simulink model "RobotBody"  (R2024b)
settings: Solver=VariableStepAuto  StartTime=0.0  StopTime=5  RelTol=1e-3
values from neighbouring files (symbols this model uses):
  N = 20    [Init.m]
  s = U_weight*eye(InputNum)    [Init.m]
undefined symbols (not defined in the file or in its folder): DiscIntNeverNeededParam, X, Y, Z
libraries: sm_lib x306, nesl_utility x75, slpidlib x6, SignalEditorBlockLib x1
(part 1 of 7)
settings Model: Creator=Rengar  LastModifiedBy=ASUS
settings RTWCC: GPUComputeCapability=3.5

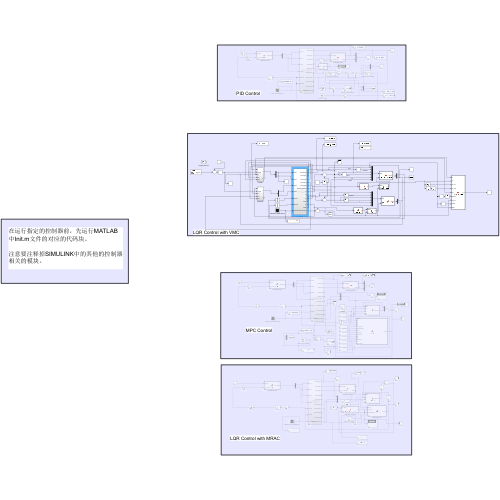
[thumbnail: Simulink's stored preview of the top-level diagram]
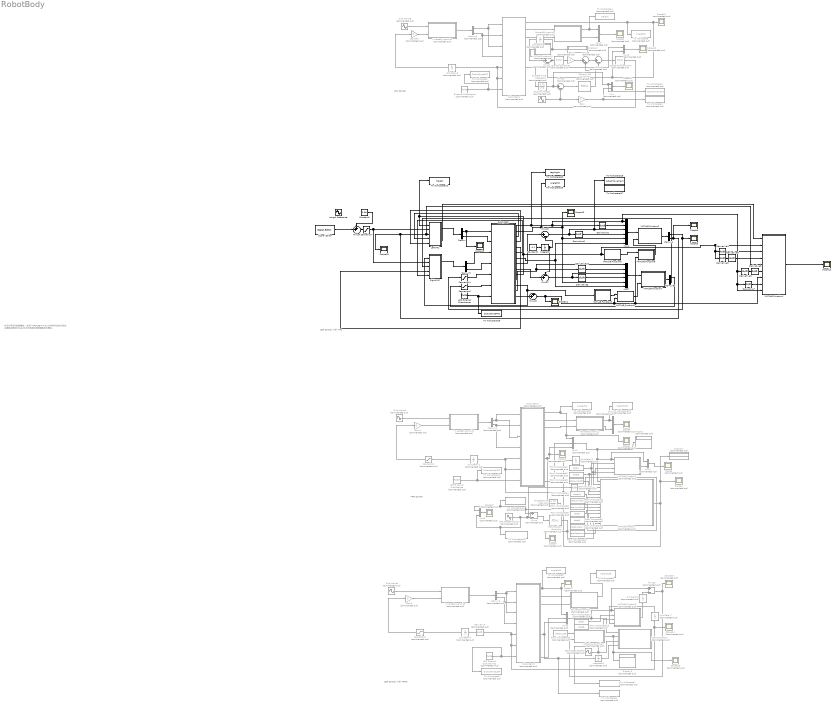
== system RobotBody ==
  note: 在运行指定的控制器前，先运行MATLAB中Init.m文件的对应的代码块。
      |
      | 注意要注释掉SIMULINK中的其他的控制器相关的模块。
  note: PID Control
  note: LQR Control with VMC
  note: MPC Control
  note: LQR Control with MRAC
  Adaptive controller1 : MATLAB Function  Commented=on  TreatAsAtomicUnit=on  SystemSampleTime=0.001
  Angle PID Controller : slpidlib/PID Controller  Commented=on  Controller=PID  Form=Parallel  TimeDomain=Continuous-time  UseExternalTs=off  SampleTime=-1  IntegratorMethod=Forward Euler  FilterMethod=Forward Euler  ControllerParametersSource=internal  P=1000  I=0  UseKiTs=off  D=500  UseExternalDerivativeSource=off  N=100  UseFilter=on  TunerSelectOption=Transfer Function Based (PID Tuner App)  InitialConditionSource=internal  InitialConditionForIntegrator=0  InitialConditionForFilter=0  DifferentiatorICPrevScaledInput=0  ExternalReset=none  TrackingMode=off  Kt=1  LimitOutput=off  SatLimitsSource=internal  UpperSaturationLimit=inf  LowerSaturationLimit=-inf  LinearizeAsGain=on  AntiWindupMode=none  Kb=1  LimitIntegrator=off  UpperIntegratorSaturationLimit=inf  LowerIntegratorSaturationLimit=-inf  POutMin=[]  POutMax=[]  IOutMin=[]  IOutMax=[]  DOutMin=[]  DOutMax=[]  NOutMin=[]  NOutMax=[]  SumOutMin=[]  SumOutMax=[]  SaturationOutMin=[]  SaturationOutMax=[]  PParamMin=[]  PParamMax=[]  IParamMin=[]  IParamMax=[]  DParamMin=[]  DParamMax=[]  NParamMin=[]  NParamMax=[]  KbParamMin=[]  KbParamMax=[]  KtParamMin=[]  KtParamMax=[]  KbOutMin=[]  KbOutMax=[]  KtOutMin=[]  KtOutMax=[]  IntegratorOutMin=[]  IntegratorOutMax=[]  FilterOutMin=[]  FilterOutMax=[]  SumI1OutMin=[]  SumI1OutMax=[]  SumI2OutMin=[]  SumI2OutMax=[]  SumI3OutMin=[]  SumI3OutMax=[]  SumI4OutMin=[]  SumI4OutMax=[]  SumDOutMin=[]  SumDOutMax=[]  DifferentiatorOutMin=[]  DifferentiatorOutMax=[]  FilterDiffOutCoefMin=[]  FilterDiffOutCoefMax=[]  ReciprocalOutMin=[]  ReciprocalOutMax=[]  SumDenOutMin=[]  SumDenOutMax=[]  SumNumOutMin=[]  SumNumOutMax=[]  DivideOutMin=[]  DivideOutMax=[]  UdiffTsProdOutMin=[]  UdiffTsProdOutMax=[]  NTsProdOutMin=[]  NTsProdOutMax=[]  UintegralTsProdOutMin=[]  UintegralTsProdOutMax=[]  UngainTsProdOutMin=[]  UngainTsProdOutMax=[]  ClampingZeroOutDataTypeStr=Inherit: Inherit via back propagation  ClampingZeroOutMin=[]  ClampingZeroOutMax=[]  FilterDenConstantOutDataTypeStr=Inherit: Inherit via back propagation  FilterDenConstantOutMin=[]  FilterDenConstantOutMax=[]  PCopyOutDataTypeStr=Inherit: Inherit via back propagation  PCopyOutMin=[]  PCopyOutMax=[]  NCopyOutDataTypeStr=Inherit: Inherit via back propagation  NCopyOutMin=[]  NCopyOutMax=[]  IntegratorContinuousStateAttributes=''  IntegratorStateMustResolveToSignalObject=off  IntegratorRTWStateStorageClass=Auto  FilterContinuousStateAttributes=''  FilterStateMustResolveToSignalObject=off  FilterRTWStateStorageClass=Auto  ParallelPVariant=InternalParameters  IdealPVariant=Disabled  IVariant=InternalParameters  DVariant=InternalParameters  IntegratorVariant=Continuous  SatVariant=Disabled  AWVariant=Passthrough  PCopyVariant=Disabled  TRVariant=Disabled  FdbkBlocksVariant=Forward  IdealPFdbkVariant=Disabled  SatFdbkVariant=Disabled  DerivativeFilterVariant=ContFilter  NVariant=InternalParameters  NCopyVariant=Disabled  FilterICVariant=InternalICsFilter  IntegratorICVariant=InternalICs  ExternalResetVariant=Disabled  TRSumVariant=Passthrough  SumFdbkVariant=Disabled  SumVariant=Sum_PID  TsampFilterVariant=InternalTs  TsampNgainVariant=Passthrough  TsampIntegralVariant=Disabled_SignalSpec  ExternalSaturationOutDataTypeStr=Inherit: Same as second input  DerivativeSourceVariant=ErrorSignal  PreIntVariant=InternalPreInt
  Constant1 : Constant  Value=0.06
  Constant2 : Constant  Value=-1.1
  Demux{,4..6} (4 alike) : Demux  Outputs=2
  Demux1 : Demux  Commented=on  Outputs=2
  Demux2 : Demux  Commented=on  Outputs=2
  Demux3 : Demux  Commented=on  Outputs=2
  Derivative : Derivative  Commented=on
  Derivative{1..10} (10 alike) : Derivative
  Derivative11 : Derivative  Commented=on
  Discrete-Time Integrator : DiscreteIntegrator  Commented=on  SampleTime=0.001  ICPrevOutput=DiscIntNeverNeededParam  ICPrevScaledInput=DiscIntNeverNeededParam
  Discrete-Time Integrator1 : DiscreteIntegrator  Commented=on  SampleTime=0.001  ICPrevOutput=DiscIntNeverNeededParam  ICPrevScaledInput=DiscIntNeverNeededParam
  Display{,1..3} (4 alike) : Display  Commented=on
  External Disturbance : DiscretePulseGenerator  Commented=on  PulseType=Time based  Amplitude=0  Period=10  PhaseDelay=2
  ForwardDynamic1 : MATLAB Function  Commented=on  TreatAsAtomicUnit=on  SystemSampleTime=0.001
  ForwardDynamic2 : MATLAB Function  Commented=on  TreatAsAtomicUnit=on  SystemSampleTime=0.01
  ForwardDynamic3 : MATLAB Function  Commented=on  TreatAsAtomicUnit=on  SystemSampleTime=0.001
  From Workspace1 : FromWorkspace  Commented=on  VariableName=dataA  SampleTime=-1  Interpolate=off  ZeroCross=off  OutputAfterFinalValue=Holding final value
  From Workspace10 : FromWorkspace  Commented=on  VariableName=dataStateNum  SampleTime=-1  Interpolate=off  ZeroCross=off  OutputAfterFinalValue=Holding final value
  From Workspace13 : FromWorkspace  Commented=on  VariableName=dataK_LQR
  From Workspace14 : FromWorkspace  Commented=on  VariableName=dataA  SampleTime=-1  Interpolate=off  ZeroCross=off  OutputAfterFinalValue=Holding final value
  From Workspace15 : FromWorkspace  Commented=on  VariableName=dataB  SampleTime=-1  Interpolate=off  ZeroCross=off  OutputAfterFinalValue=Holding final value
  From Workspace2 : FromWorkspace  Commented=on  VariableName=dataB  SampleTime=-1  Interpolate=off  ZeroCross=off  OutputAfterFinalValue=Holding final value
  From Workspace3 : FromWorkspace  Commented=on  VariableName=dataU_weight  SampleTime=-1  Interpolate=off  ZeroCross=off  OutputAfterFinalValue=Holding final value
  From Workspace4 : FromWorkspace  Commented=on  VariableName=dataPhi  SampleTime=-1  Interpolate=off  ZeroCross=off  OutputAfterFinalValue=Holding final value
  From Workspace5 : FromWorkspace  Commented=on  VariableName=dataInputNum  SampleTime=-1  Interpolate=off  ZeroCross=off  OutputAfterFinalValue=Holding final value
  From Workspace6 : FromWorkspace  Commented=on  VariableName=dataLambda  SampleTime=-1  Interpolate=off  ZeroCross=off  OutputAfterFinalValue=Holding final value
  From Workspace7 : FromWorkspace  Commented=on  VariableName=dataQ  SampleTime=-1  Interpolate=off  ZeroCross=off  OutputAfterFinalValue=Holding final value
  From Workspace8 : FromWorkspace  Commented=on  VariableName=dataN  SampleTime=-1  Interpolate=off  ZeroCross=off  OutputAfterFinalValue=Holding final value
  From Workspace9 : FromWorkspace  Commented=on  VariableName=dataS_Matrix  SampleTime=-1  Interpolate=off  ZeroCross=off  OutputAfterFinalValue=Holding final value
  Gain : Gain  Commented=on
  Gain1 : Gain  Commented=on  Gain=0
  Gain3 : Gain  Commented=on  Gain=-1
  Gain4 : Gain  Commented=on  Gain=0
  Integrator : Integrator
  Integrator1 : Integrator  Commented=on
  InverseDynanmic1 : MATLAB Function  Commented=on  TreatAsAtomicUnit=on
  InverseDynanmic2 : MATLAB Function  Commented=on  TreatAsAtomicUnit=on  SystemSampleTime=0.01
  InverseDynanmic3 : MATLAB Function  Commented=on  TreatAsAtomicUnit=on
  LQR Controller1 : MATLAB Function  Commented=on  TreatAsAtomicUnit=on  SystemSampleTime=0.001
  LQR External Disturbance : DiscretePulseGenerator  PulseType=Time based  Amplitude=0  Period=10  PhaseDelay=2
  LQR External Disturbance1 : DiscretePulseGenerator  Commented=on  PulseType=Time based  Amplitude=0  Period=10  PhaseDelay=2
  LQR Target Speed1 : Sin  Commented=on  Amplitude=0  Frequency=0.628  SampleTime=0
  LeftVMC : Subsystem
  Leg Gain : Gain  Commented=on  Gain=0
  Length Reference : Sin  Amplitude=0  Bias=0.076  Frequency=0.628  SampleTime=0
  MATLAB Function : MATLAB Function  Commented=on  TreatAsAtomicUnit=on  SystemSampleTime=0.001
  MATLAB Function1 : MATLAB Function  Commented=on  TreatAsAtomicUnit=on
  MATLAB Function10 : MATLAB Function  Commented=on  TreatAsAtomicUnit=on  SystemSampleTime=0.001
  MATLAB Function2 : MATLAB Function  TreatAsAtomicUnit=on
  MATLAB Function3 : MATLAB Function  Commented=on  TreatAsAtomicUnit=on  SystemSampleTime=0.001
  MATLAB Function4 : MATLAB Function  TreatAsAtomicUnit=on
  MATLAB Function5 : MATLAB Function  TreatAsAtomicUnit=on
  MATLAB Function6 : MATLAB Function  TreatAsAtomicUnit=on
  MATLAB Function7 : MATLAB Function  TreatAsAtomicUnit=on
  MATLAB Function8 : MATLAB Function  TreatAsAtomicUnit=on
  MATLAB Function9 : MATLAB Function  TreatAsAtomicUnit=on
  MPC External Disturbance : DiscretePulseGenerator  Commented=on  PulseType=Time based  Period=5  PhaseDelay=1
  MPC Position Controller : slpidlib/PID Controller  Commented=on  Controller=PD  Form=Parallel  TimeDomain=Discrete-time  UseExternalTs=off  SampleTime=-1  IntegratorMethod=Forward Euler  FilterMethod=Forward Euler  ControllerParametersSource=internal  P=5  I=0.1  UseKiTs=off  D=0.3  UseExternalDerivativeSource=off  N=10  UseFilter=on  TunerSelectOption=Transfer Function Based (PID Tuner App)  InitialConditionSource=internal  InitialConditionForIntegrator=0  InitialConditionForFilter=0  DifferentiatorICPrevScaledInput=0  ExternalReset=none  TrackingMode=off  Kt=1  LimitOutput=on  SatLimitsSource=internal  UpperSaturationLimit=30  LowerSaturationLimit=-30  LinearizeAsGain=on  AntiWindupMode=none  Kb=1  LimitIntegrator=off  UpperIntegratorSaturationLimit=inf  LowerIntegratorSaturationLimit=-inf  POutMin=[]  POutMax=[]  IOutMin=[]  IOutMax=[]  DOutMin=[]  DOutMax=[]  NOutMin=[]  NOutMax=[]  SumOutMin=[]  SumOutMax=[]  SaturationOutMin=[]  SaturationOutMax=[]  PParamMin=[]  PParamMax=[]  IParamMin=[]  IParamMax=[]  DParamMin=[]  DParamMax=[]  NParamMin=[]  NParamMax=[]  KbParamMin=[]  KbParamMax=[]  KtParamMin=[]  KtParamMax=[]  KbOutMin=[]  KbOutMax=[]  KtOutMin=[]  KtOutMax=[]  IntegratorOutMin=[]  IntegratorOutMax=[]  FilterOutMin=[]  FilterOutMax=[]  SumI1OutMin=[]  SumI1OutMax=[]  SumI2OutMin=[]  SumI2OutMax=[]  SumI3OutMin=[]  SumI3OutMax=[]  SumI4OutMin=[]  SumI4OutMax=[]  SumDOutMin=[]  SumDOutMax=[]  DifferentiatorOutMin=[]  DifferentiatorOutMax=[]  FilterDiffOutCoefMin=[]  FilterDiffOutCoefMax=[]  ReciprocalOutMin=[]  ReciprocalOutMax=[]  SumDenOutMin=[]  SumDenOutMax=[]  SumNumOutMin=[]  SumNumOutMax=[]  DivideOutMin=[]  DivideOutMax=[]  UdiffTsProdOutMin=[]  UdiffTsProdOutMax=[]  NTsProdOutMin=[]  NTsProdOutMax=[]  UintegralTsProdOutMin=[]  UintegralTsProdOutMax=[]  UngainTsProdOutMin=[]  UngainTsProdOutMax=[]  ClampingZeroOutDataTypeStr=Inherit: Inherit via back propagation  ClampingZeroOutMin=[]  ClampingZeroOutMax=[]  FilterDenConstantOutDataTypeStr=Inherit: Inherit via back propagation  FilterDenConstantOutMin=[]  FilterDenConstantOutMax=[]  PCopyOutDataTypeStr=Inherit: Inherit via back propagation  PCopyOutMin=[]  PCopyOutMax=[]  NCopyOutDataTypeStr=Inherit: Inherit via back propagation  NCopyOutMin=[]  NCopyOutMax=[]  IntegratorContinuousStateAttributes=''  IntegratorStateMustResolveToSignalObject=off  IntegratorRTWStateStorageClass=Auto  FilterContinuousStateAttributes=''  FilterStateMustResolveToSignalObject=off  FilterRTWStateStorageClass=Auto  ParallelPVariant=InternalParameters  IdealPVariant=Disabled  IVariant=Disabled  DVariant=InternalParameters  IntegratorVariant=Disabled  SatVariant=Enabled  AWVariant=Disabled  PCopyVariant=Disabled  TRVariant=Disabled  FdbkBlocksVariant=Forward  IdealPFdbkVariant=Disabled  SatFdbkVariant=Disabled  DerivativeFilterVariant=ForwardEulerFilter  NVariant=InternalParameters  NCopyVariant=Disabled  FilterICVariant=InternalICsFilter  IntegratorICVariant=Disabled  ExternalResetVariant=Disabled  TRSumVariant=Passthrough  SumFdbkVariant=Disabled  SumVariant=Sum_PD  TsampFilterVariant=InternalTs  TsampNgainVariant=Passthrough  TsampIntegralVariant=Disabled_SignalSpec  ExternalSaturationOutDataTypeStr=Inherit: Same as second input  DerivativeSourceVariant=ErrorSignal  PreIntVariant=InternalPreInt
  MPC Target Position : Sin  Commented=on  Amplitude=0  Frequency=0.628  SampleTime=0
  Minus : Sum  Commented=on  Inputs=+-
  Minus1 : Sum  Commented=on  Inputs=|+-
  Minus2 : Sum  Commented=on  Inputs=|+-
  Minus3 : Sum  Inputs=++|
  Minus4 : Sum  Inputs=++|
  Minus5 : Sum  Commented=on  Inputs=|+-
  Minus6 : Sum  Commented=on  Inputs=|++
  Minus7 : Sum  Inputs=-+|
  Minus8 : Sum  Commented=on  Inputs=+-
  Minus9 : Sum  Inputs=|+-
  Mux{,2,4..6,9} (6 alike) : Mux  Commented=on  Inputs=2
  Mux1 : Mux  Inputs=6
  Mux3 : Mux  Commented=on  Inputs=3
  Mux7 : Mux  Inputs=6
  Mux8 : Mux  Commented=on  Inputs=3
  Position PID Controller : slpidlib/PID Controller  Commented=on  Controller=PID  Form=Parallel  TimeDomain=Continuous-time  UseExternalTs=off  SampleTime=-1  IntegratorMethod=Forward Euler  FilterMethod=Forward Euler  ControllerParametersSource=internal  P=5  I=0  UseKiTs=off  D=80  UseExternalDerivativeSource=off  N=100  UseFilter=on  TunerSelectOption=Transfer Function Based (PID Tuner App)  InitialConditionSource=internal  InitialConditionForIntegrator=0  InitialConditionForFilter=0  DifferentiatorICPrevScaledInput=0  ExternalReset=none  TrackingMode=off  Kt=1  LimitOutput=on  SatLimitsSource=internal  UpperSaturationLimit=100  LowerSaturationLimit=-100  LinearizeAsGain=on  AntiWindupMode=none  Kb=1  LimitIntegrator=off  UpperIntegratorSaturationLimit=inf  LowerIntegratorSaturationLimit=-inf  POutMin=[]  POutMax=[]  IOutMin=[]  IOutMax=[]  DOutMin=[]  DOutMax=[]  NOutMin=[]  NOutMax=[]  SumOutMin=[]  SumOutMax=[]  SaturationOutMin=[]  SaturationOutMax=[]  PParamMin=[]  PParamMax=[]  IParamMin=[]  IParamMax=[]  DParamMin=[]  DParamMax=[]  NParamMin=[]  NParamMax=[]  KbParamMin=[]  KbParamMax=[]  KtParamMin=[]  KtParamMax=[]  KbOutMin=[]  KbOutMax=[]  KtOutMin=[]  KtOutMax=[]  IntegratorOutMin=[]  IntegratorOutMax=[]  FilterOutMin=[]  FilterOutMax=[]  SumI1OutMin=[]  SumI1OutMax=[]  SumI2OutMin=[]  SumI2OutMax=[]  SumI3OutMin=[]  SumI3OutMax=[]  SumI4OutMin=[]  SumI4OutMax=[]  SumDOutMin=[]  SumDOutMax=[]  DifferentiatorOutMin=[]  DifferentiatorOutMax=[]  FilterDiffOutCoefMin=[]  FilterDiffOutCoefMax=[]  ReciprocalOutMin=[]  ReciprocalOutMax=[]  SumDenOutMin=[]  SumDenOutMax=[]  SumNumOutMin=[]  SumNumOutMax=[]  DivideOutMin=[]  DivideOutMax=[]  UdiffTsProdOutMin=[]  UdiffTsProdOutMax=[]  NTsProdOutMin=[]  NTsProdOutMax=[]  UintegralTsProdOutMin=[]  UintegralTsProdOutMax=[]  UngainTsProdOutMin=[]  UngainTsProdOutMax=[]  ClampingZeroOutDataTypeStr=Inherit: Inherit via back propagation  ClampingZeroOutMin=[]  ClampingZeroOutMax=[]  FilterDenConstantOutDataTypeStr=Inherit: Inherit via back propagation  FilterDenConstantOutMin=[]  FilterDenConstantOutMax=[]  PCopyOutDataTypeStr=Inherit: Inherit via back propagation  PCopyOutMin=[]  PCopyOutMax=[]  NCopyOutDataTypeStr=Inherit: Inherit via back propagation  NCopyOutMin=[]  NCopyOutMax=[]  IntegratorContinuousStateAttributes=''  IntegratorStateMustResolveToSignalObject=off  IntegratorRTWStateStorageClass=Auto  FilterContinuousStateAttributes=''  FilterStateMustResolveToSignalObject=off  FilterRTWStateStorageClass=Auto  ParallelPVariant=InternalParameters  IdealPVariant=Disabled  IVariant=InternalParameters  DVariant=InternalParameters  IntegratorVariant=Continuous  SatVariant=Enabled  AWVariant=Passthrough  PCopyVariant=Disabled  TRVariant=Disabled  FdbkBlocksVariant=Forward  IdealPFdbkVariant=Disabled  SatFdbkVariant=Disabled  DerivativeFilterVariant=ContFilter  NVariant=InternalParameters  NCopyVariant=Disabled  FilterICVariant=InternalICsFilter  IntegratorICVariant=InternalICs  ExternalResetVariant=Disabled  TRSumVariant=Passthrough  SumFdbkVariant=Disabled  SumVariant=Sum_PID  TsampFilterVariant=InternalTs  TsampNgainVariant=Passthrough  TsampIntegralVariant=Disabled_SignalSpec  ExternalSaturationOutDataTypeStr=Inherit: Same as second input  DerivativeSourceVariant=ErrorSignal  PreIntVariant=InternalPreInt
  Position Target : Sin  Commented=on  Amplitude=0  Frequency=0.628  SampleTime=0
  RightVMC : Subsystem
  Saturation1 : Saturate  Commented=on  UpperLimit=1  LowerLimit=-1
  Saturation2 : Saturate  Commented=on  UpperLimit=1  LowerLimit=-1
  Saturation4 : Saturate  ZeroCross=off
  Saturation6 : Saturate  ZeroCross=off
  Saturation7 : Saturate  UpperLimit=1  LowerLimit=0.06  ZeroCross=off
  Scope{1..2,4..8,10,14..17,20..22} (15 alike) : Scope  Commented=on
  Scope{3,9,11..13,18..19} (7 alike) : Scope
  Signal Editor : SignalEditorBlockLib/Signal Editor  FileName=JumpLeg.mat  ActiveScenario=Scenario  ActiveSignal=Signal 1  IsBus=off  OutputBusObjectStr=Bus: BusObject  SampleTime=0  Interpolate=off  ZeroCross=off  OutputAfterFinalValue=Setting to zero  Unit=inherit  PreserveSignalName=on  ApplySigPropsToAllScenarios=on  ApplySigPropsToAllSignals=off
  Sine Wave3 : Sin  Commented=on  Amplitude=0  Bias=50  Frequency=0.628  SampleTime=0
  Sine Wave4 : Sin  Commented=on  Amplitude=0  Bias=50  Frequency=0.628  SampleTime=0
  Sine Wave5 : Sin  Commented=on  Amplitude=0  Bias=50  Frequency=0.628  SampleTime=0
  Speed PID Controller : slpidlib/PID Controller  Commented=on  Controller=PID  Form=Parallel  TimeDomain=Continuous-time  UseExternalTs=off  SampleTime=-1  IntegratorMethod=Forward Euler  FilterMethod=Forward Euler  ControllerParametersSource=internal  P=1  I=0.2  UseKiTs=off  D=0  UseExternalDerivativeSource=off  N=100  UseFilter=on  TunerSelectOption=Transfer Function Based (PID Tuner App)  InitialConditionSource=internal  InitialConditionForIntegrator=0  InitialConditionForFilter=0  DifferentiatorICPrevScaledInput=0  ExternalReset=none  TrackingMode=off  Kt=1  LimitOutput=off  SatLimitsSource=internal  UpperSaturationLimit=inf  LowerSaturationLimit=-inf  LinearizeAsGain=on  AntiWindupMode=none  Kb=1  LimitIntegrator=off  UpperIntegratorSaturationLimit=inf  LowerIntegratorSaturationLimit=-inf  POutMin=[]  POutMax=[]  IOutMin=[]  IOutMax=[]  DOutMin=[]  DOutMax=[]  NOutMin=[]  NOutMax=[]  SumOutMin=[]  SumOutMax=[]  SaturationOutMin=[]  SaturationOutMax=[]  PParamMin=[]  PParamMax=[]  IParamMin=[]  IParamMax=[]  DParamMin=[]  DParamMax=[]  NParamMin=[]  NParamMax=[]  KbParamMin=[]  KbParamMax=[]  KtParamMin=[]  KtParamMax=[]  KbOutMin=[]  KbOutMax=[]  KtOutMin=[]  KtOutMax=[]  IntegratorOutMin=[]  IntegratorOutMax=[]  FilterOutMin=[]  FilterOutMax=[]  SumI1OutMin=[]  SumI1OutMax=[]  SumI2OutMin=[]  SumI2OutMax=[]  SumI3OutMin=[]  SumI3OutMax=[]  SumI4OutMin=[]  SumI4OutMax=[]  SumDOutMin=[]  SumDOutMax=[]  DifferentiatorOutMin=[]  DifferentiatorOutMax=[]  FilterDiffOutCoefMin=[]  FilterDiffOutCoefMax=[]  ReciprocalOutMin=[]  ReciprocalOutMax=[]  SumDenOutMin=[]  SumDenOutMax=[]  SumNumOutMin=[]  SumNumOutMax=[]  DivideOutMin=[]  DivideOutMax=[]  UdiffTsProdOutMin=[]  UdiffTsProdOutMax=[]  NTsProdOutMin=[]  NTsProdOutMax=[]  UintegralTsProdOutMin=[]  UintegralTsProdOutMax=[]  UngainTsProdOutMin=[]  UngainTsProdOutMax=[]  ClampingZeroOutDataTypeStr=Inherit: Inherit via back propagation  ClampingZeroOutMin=[]  ClampingZeroOutMax=[]  FilterDenConstantOutDataTypeStr=Inherit: Inherit via back propagation  FilterDenConstantOutMin=[]  FilterDenConstantOutMax=[]  PCopyOutDataTypeStr=Inherit: Inherit via back propagation  PCopyOutMin=[]  PCopyOutMax=[]  NCopyOutDataTypeStr=Inherit: Inherit via back propagation  NCopyOutMin=[]  NCopyOutMax=[]  IntegratorContinuousStateAttributes=''  IntegratorStateMustResolveToSignalObject=off  IntegratorRTWStateStorageClass=Auto  FilterContinuousStateAttributes=''  FilterStateMustResolveToSignalObject=off  FilterRTWStateStorageClass=Auto  ParallelPVariant=InternalParameters  IdealPVariant=Disabled  IVariant=InternalParameters  DVariant=InternalParameters  IntegratorVariant=Continuous  SatVariant=Disabled  AWVariant=Passthrough  PCopyVariant=Disabled  TRVariant=Disabled  FdbkBlocksVariant=Forward  IdealPFdbkVariant=Disabled  SatFdbkVariant=Disabled  DerivativeFilterVariant=ContFilter  NVariant=InternalParameters  NCopyVariant=Disabled  FilterICVariant=InternalICsFilter  IntegratorICVariant=InternalICs  ExternalResetVariant=Disabled  TRSumVariant=Passthrough  SumFdbkVariant=Disabled  SumVariant=Sum_PID  TsampFilterVariant=InternalTs  TsampNgainVariant=Passthrough  TsampIntegralVariant=Disabled_SignalSpec  ExternalSaturationOutDataTypeStr=Inherit: Same as second input  DerivativeSourceVariant=ErrorSignal  PreIntVariant=InternalPreInt
  Subsystem : Subsystem
  Subsystem1 : Subsystem  Commented=on
  Subsystem3 : Subsystem  Commented=on
  Subsystem4 : Subsystem  Commented=on
  To Workspace : ToWorkspace  Commented=on  VariableName=AnglePID  SaveFormat=Timeseries  SampleTime=-1
  To Workspace1 : ToWorkspace  Commented=on  VariableName=DisturbancePID  SaveFormat=Timeseries  SampleTime=-1
  To Workspace10 : ToWorkspace  Commented=on  VariableName=AngleMPC  SaveFormat=Timeseries  SampleTime=-1
  To Workspace11 : ToWorkspace  Commented=on  VariableName=ActualMovementMPC  SaveFormat=Timeseries  SampleTime=-1
  To Workspace12 : ToWorkspace  Commented=on  VariableName=ReferenceMovementMPC  SaveFormat=Timeseries  SampleTime=-1
  To Workspace13 : ToWorkspace  Commented=on  VariableName=HeightMPC  SaveFormat=Timeseries  SampleTime=-1
  To Workspace14 : ToWorkspace  Commented=on  VariableName=DisturbanceMPC  SaveFormat=Timeseries  SampleTime=-1
  To Workspace15 : ToWorkspace  VariableName=Height  SaveFormat=Timeseries  SampleTime=-1
  To Workspace16 : ToWorkspace  VariableName=ActualMovement  SaveFormat=Timeseries  SampleTime=-1
  To Workspace17 : ToWorkspace  VariableName=ReferenceMovement  SaveFormat=Timeseries  SampleTime=-1
  To Workspace18 : ToWorkspace  VariableName=DisturbancePID  SaveFormat=Timeseries  SampleTime=-1
  To Workspace19 : ToWorkspace  VariableName=AnglePID  SaveFormat=Timeseries  SampleTime=-1
  To Workspace2 : ToWorkspace  Commented=on  VariableName=ActualMovement  SaveFormat=Timeseries  SampleTime=-1
  To Workspace20 : ToWorkspace  VariableName=LegAngle  SaveFormat=Timeseries  SampleTime=-1
  To Workspace3 : ToWorkspace  Commented=on  VariableName=ReferenceMovement  SaveFormat=Timeseries  SampleTime=-1
  To Workspace4 : ToWorkspace  Commented=on  VariableName=Height  SaveFormat=Timeseries  SampleTime=-1
  To Workspace5 : ToWorkspace  Commented=on  VariableName=AngleLQR  SaveFormat=Timeseries  SampleTime=-1
  To Workspace6 : ToWorkspace  Commented=on  VariableName=ActualMovementLQR  SaveFormat=Timeseries  SampleTime=-1
  To Workspace7 : ToWorkspace  Commented=on  VariableName=ReferenceMovementLQR  SaveFormat=Timeseries  SampleTime=-1
  To Workspace8 : ToWorkspace  Commented=on  VariableName=DisturbanceLQR  SaveFormat=Timeseries  SampleTime=-1
  To Workspace9 : ToWorkspace  Commented=on  VariableName=HeightLQR  SaveFormat=Timeseries  SampleTime=-1
  Unit Delay{1,3..5} (4 alike) : UnitDelay  Commented=on  SampleTime=-1  HasFrameUpgradeWarning=on
  Unit Delay2 : UnitDelay  Commented=on  SampleTime=0.001  HasFrameUpgradeWarning=on
  Unit Delay7 : UnitDelay  Commented=on  SampleTime=0.001  HasFrameUpgradeWarning=on
  Unit Delay8 : UnitDelay  Commented=on  SampleTime=0.001  HasFrameUpgradeWarning=on
  wires:
  Demux/1 -> Subsystem/1(Joint1), Scope19/1
  Demux/2 -> Subsystem/2(Joint2)
  Subsystem/2(JointAngle1) -> LeftVMC/4(Phi1)
  Subsystem/3(JointAngle2) -> LeftVMC/5(Phi4)
  Subsystem/1(RobotAngle) -> To Workspace19/1, Mux1/5, Mux7/5, Scope13/1  "Phi"
  Unit Delay1/1 -> Saturation1/1
  Gain1/1 -> InverseDynanmic1/2(TargetTheta)
  Sine Wave3/1 -> InverseDynanmic1/1(TargetL)
  Saturation1/1 -> Gain1/1
  Subsystem1/10(RobotAngleSpeed) -> Mux3/2
  Demux2/2 -> Subsystem1/4(Joint4), Subsystem1/2(Joint2)
  ForwardDynamic1/2(Theta) -> Mux2/2
  Subsystem1/3(JointAngle2) -> ForwardDynamic1/2(JointAngle2)
  Mux2/1 -> Scope2/1
  ForwardDynamic1/1(L) -> To Workspace13/1, Mux2/1
  Demux2/1 -> Subsystem1/1(Joint1), Subsystem1/3(Joint3)
  Subsystem1/2(JointAngle1) -> ForwardDynamic1/1(JointAngle1)
  Subsystem1/7(WheelSpeed1) -> Discrete-Time Integrator/1, Scope5/1, Mux3/3
  InverseDynanmic1/1(JointAngle) -> Demux2/1
  Mux3/1 -> Mux4/1, MATLAB Function1/1(State), MATLAB Function/1(State), Display/1
  MATLAB Function/1(Torque) -> Display1/1, Scope4/1, Unit Delay2/1, Subsystem1/6(Wheel2), Subsystem1/5(Wheel1), Unit Delay1/1
  Unit Delay2/1 -> MATLAB Function/2(U), MATLAB Function1/4(U)
  Derivative11/1 -> MATLAB Function/6(TargetSpeed)
  From Workspace2/1 -> MATLAB Function1/3(B), MATLAB Function/4(B)
  From Workspace1/1 -> MATLAB Function1/2(A), MATLAB Function/3(A)
  From Workspace3/1 -> MATLAB Function/5(U_weight)
  From Workspace4/1 -> MATLAB Function/7(Phi)
  From Workspace6/1 -> MATLAB Function/8(Lambda)
  From Workspace5/1 -> MATLAB Function/9(InputNum)
  From Workspace8/1 -> MATLAB Function/10(N)
  From Workspace7/1 -> MATLAB Function/11(Q)
  From Workspace9/1 -> MATLAB Function/12(S_Matrix)
  MPC External Disturbance/1 -> Subsystem1/7(ExternalForce), To Workspace14/1
  LQR External Disturbance/1 -> To Workspace18/1, Subsystem/7(ExternalForce)
  MATLAB Function1/1(State_hat) -> Mux4/2
  Mux4/1 -> Scope6/1
  From Workspace10/1 -> MATLAB Function/14(StateNum)
  Subsystem1/1(RobotAngle) -> Mux3/1, Scope1/1, To Workspace10/1
  MPC Position Controller/1 -> MATLAB Function/13(X), Scope7/1
  Discrete-Time Integrator/1 -> Mux9/1, To Workspace11/1, Minus/1
  Minus/1 -> MPC Position Controller/1
  MPC Target Position/1 -> Derivative11/1, Minus/2, To Workspace12/1, Mux9/2
  InverseDynanmic2/1(JointAngle) -> Demux3/1
  Demux3/1 -> Subsystem4/1(Joint1), Subsystem4/3(Joint3)
  Demux3/2 -> Subsystem4/4(Joint4), Subsystem4/2(Joint2)
  ForwardDynamic2/1(L) -> To Workspace4/1, Mux5/1
  ForwardDynamic2/2(Theta) -> Mux5/2
  Mux5/1 -> Scope8/1
  Sine Wave5/1 -> InverseDynanmic2/1(TargetL)
  Leg Gain/1 -> InverseDynanmic2/2(TargetTheta)
  Minus1/1 -> MATLAB Function10/1(Error), Angle PID Controller/1
  Subsystem4/2(JointAngle1) -> ForwardDynamic2/1(JointAngle1)
  Subsystem4/3(JointAngle2) -> ForwardDynamic2/2(JointAngle2)
  Subsystem4/1(RobotAngle) -> Scope20/1, Mux6/2, Minus1/2, To Workspace/1
  Minus2/1 -> Speed PID Controller/1
  Subsystem4/7(WheelSpeed1) -> Discrete-Time Integrator1/1, Mux6/1, Minus2/2
  Unit Delay3/1 -> Leg Gain/1
  Mux6/1 -> Scope10/1
  External Disturbance/1 -> Subsystem4/7(ExternalForce), To Workspace1/1
  Angle PID Controller/1 -> Gain3/1
  Discrete-Time Integrator1/1 -> To Workspace2/1, Mux/1, Minus5/1
  Position Target/1 -> Minus5/2, Gain/1
  Minus5/1 -> Position PID Controller/1
  Speed PID Controller/1 -> Subsystem4/6(Wheel2), Subsystem4/5(Wheel1), Unit Delay3/1
  Unit Delay8/1 -> Minus8/2
  Minus8/1 -> Scope15/1, Adaptive controller1/2(Error)
  From Workspace13/1 -> Adaptive controller1/1(K_LQR)
  LQR External Disturbance1/1 -> To Workspace8/1, Subsystem3/7(ExternalForce)
  LQR Controller1/1(Torque) -> Derivative/1, Subsystem3/5(Wheel1), Subsystem3/6(Wheel2), Scope14/1, Unit Delay7/1
  Unit Delay7/1 -> MATLAB Function3/4(U)
  Subsystem3/7(WheelSpeed1) -> Mux8/3, Integrator1/1, To Workspace6/1
  From Workspace15/1 -> MATLAB Function3/3(B)
  Adaptive controller1/1(K) -> LQR Controller1/2(K_LQR), Scope16/1, Display3/1
  Subsystem3/1(RobotAngle) -> To Workspace5/1, Scope17/1, Mux8/1
  LQR Target Speed1/1 -> To Workspace7/1, LQR Controller1/3(TargetSpeed)
  Mux8/1 -> LQR Controller1/1(State), Minus8/1, MATLAB Function3/1(State)
  From Workspace14/1 -> MATLAB Function3/2(A)
  MATLAB Function3/1(State_hat) -> Unit Delay8/1
  Subsystem3/10(RobotAngleSpeed) -> Mux8/2
  Integrator1/1 -> LQR Controller1/4(X)
  Demux1/1 -> Subsystem3/3(Joint3), Subsystem3/1(Joint1)
  Demux1/2 -> Subsystem3/2(Joint2), Subsystem3/4(Joint4)
  Subsystem3/2(JointAngle1) -> ForwardDynamic3/1(JointAngle1)
  Subsystem3/3(JointAngle2) -> ForwardDynamic3/2(JointAngle2)
  Derivative1/1 -> Mux1/2  "ThetaDot"
  InverseDynanmic3/1(JointAngle) -> Demux1/1
  Saturation2/1 -> Gain4/1
  Gain4/1 -> InverseDynanmic3/2(TargetTheta)
  Sine Wave4/1 -> InverseDynanmic3/1(TargetL)
  Unit Delay4/1 -> Saturation2/1
  Demux4/1 -> Scope3/1, Saturation4/1  "T"
  Demux4/2 -> Scope9/1, Scope18/1, MATLAB Function4/5(Tp), LeftVMC/3(Tp)  "Tp"
  Mux1/1 -> MATLAB Function2/1(State)
  MATLAB Function2/1(Torque) -> Demux4/1
  Subsystem/6(RobotAngleSpeed) -> Mux7/6, Mux1/6  "PhiDot"
  Subsystem/9(L1) -> To Workspace15/1, LeftVMC/1(L), Derivative5/1, Derivative4/1, MATLAB Function4/2(L0), MATLAB Function5/1(L)  "L1"
  Subsystem/10(theta1) -> To Workspace20/1, Derivative9/1, Derivative7/1, MATLAB Function4/9(theta), Mux1/1, Derivative1/1  "Theta"
  LeftVMC/1(T) -> Demux/1
  Saturation4/1 -> Subsystem/5(Wheel1)
  Demux5/1 -> Subsystem/3(Joint3)
  Demux5/2 -> Subsystem/4(Joint4)
  Subsystem/11(L2) -> RightVMC/1(L), MATLAB Function8/1(L)  "L2"
  Mux7/1 -> MATLAB Function7/1(State)
  MATLAB Function7/1(Torque) -> Demux6/1
  Demux6/1 -> Saturation6/1
  Saturation6/1 -> Subsystem/6(Wheel2)
  Demux6/2 -> RightVMC/3(Tp)
  Subsystem/4(JointAngle3) -> RightVMC/4(Phi1)
  Subsystem/5(JointAngle4) -> RightVMC/5(Phi4)
  MATLAB Function8/1(K) -> MATLAB Function6/1(NowK)
  Minus7/1 -> Mux7/3, Derivative3/1
  Minus9/1 -> Mux1/3, To Workspace16/1, Derivative2/1  "X"
  Saturation7/1 -> RightVMC/2(TargetL), LeftVMC/2(TargetL)
  RightVMC/1(T) -> Demux5/1
  LeftVMC/2(F) -> MATLAB Function4/1(F)
  Derivative4/1 -> MATLAB Function4/3(L0_dot)
  Derivative5/1 -> Derivative6/1
  Derivative6/1 -> MATLAB Function4/4(L0_ddot)
  Derivative9/1 -> Derivative8/1
  Derivative8/1 -> MATLAB Function4/6(ddtheta)
  Derivative7/1 -> MATLAB Function4/8(dtheta)
  Minus3/1 -> Scope12/1, MATLAB Function6/2(N), MATLAB Function9/2(N), MATLAB Function4/7(ddz_M)
  MATLAB Function6/1(K) -> MATLAB Function7/2(K)
  MATLAB Function5/1(K) -> MATLAB Function9/1(NowK)
  MATLAB Function9/1(K) -> MATLAB Function2/2(K)
  Derivative3/1 -> Mux7/4  "X"
  MATLAB Function4/1(F_N) -> Scope11/1
  Subsystem/13(Acceleration) -> Minus3/2
  Minus4/1 -> Saturation7/1
  Subsystem/12(theta2) -> Mux7/1, Derivative10/1
  Derivative2/1 -> Mux1/4  "XDot"
  Derivative10/1 -> Mux7/2  "ThetaDot"
  Subsystem/7(x1) -> Minus9/1
  Subsystem/8(x2) -> Minus7/2
  Constant2/1 -> Integrator/1
  Integrator/1 -> Minus7/1, Minus9/2
  Derivative/1 -> Unit Delay4/1
  Gain3/1 -> Minus6/1
  Minus6/1 -> Minus2/1
  Mux/1 -> Scope21/1
  Gain/1 -> To Workspace3/1, Mux/2
  Position PID Controller/1 -> Minus6/2
  MATLAB Function10/1(Angle) -> Display2/1, Unit Delay5/1
  Unit Delay5/1 -> Minus1/1
  ForwardDynamic3/1(L) -> To Workspace9/1
  Mux9/1 -> Scope22/1
  Signal Editor/1 -> Minus4/2
  Constant1/1 -> Minus4/1

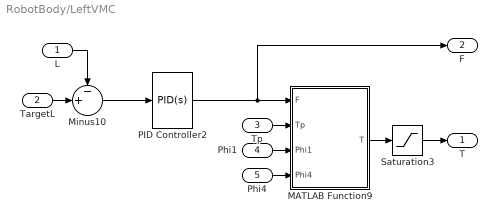
== system RobotBody/LeftVMC ==
  L : Inport
  TargetL : Inport  Port=2
  Tp : Inport  Port=3
  Phi1 : Inport  Port=4
  Phi4 : Inport  Port=5
  MATLAB Function9 : MATLAB Function  TreatAsAtomicUnit=on
  Minus10 : Sum  Inputs=-+|
  PID Controller2 : slpidlib/PID Controller  Controller=PID  Form=Parallel  TimeDomain=Continuous-time  UseExternalTs=off  SampleTime=-1  IntegratorMethod=Forward Euler  FilterMethod=Forward Euler  ControllerParametersSource=internal  P=500  I=1100  UseKiTs=off  D=50  UseExternalDerivativeSource=off  N=100  UseFilter=on  TunerSelectOption=Transfer Function Based (PID Tuner App)  InitialConditionSource=internal  InitialConditionForIntegrator=0  InitialConditionForFilter=0  DifferentiatorICPrevScaledInput=0  ExternalReset=none  TrackingMode=off  Kt=1  LimitOutput=off  SatLimitsSource=internal  UpperSaturationLimit=inf  LowerSaturationLimit=-inf  LinearizeAsGain=on  AntiWindupMode=none  Kb=1  LimitIntegrator=off  UpperIntegratorSaturationLimit=inf  LowerIntegratorSaturationLimit=-inf  POutMin=[]  POutMax=[]  IOutMin=[]  IOutMax=[]  DOutMin=[]  DOutMax=[]  NOutMin=[]  NOutMax=[]  SumOutMin=[]  SumOutMax=[]  SaturationOutMin=[]  SaturationOutMax=[]  PParamMin=[]  PParamMax=[]  IParamMin=[]  IParamMax=[]  DParamMin=[]  DParamMax=[]  NParamMin=[]  NParamMax=[]  KbParamMin=[]  KbParamMax=[]  KtParamMin=[]  KtParamMax=[]  KbOutMin=[]  KbOutMax=[]  KtOutMin=[]  KtOutMax=[]  IntegratorOutMin=[]  IntegratorOutMax=[]  FilterOutMin=[]  FilterOutMax=[]  SumI1OutMin=[]  SumI1OutMax=[]  SumI2OutMin=[]  SumI2OutMax=[]  SumI3OutMin=[]  SumI3OutMax=[]  SumI4OutMin=[]  SumI4OutMax=[]  SumDOutMin=[]  SumDOutMax=[]  DifferentiatorOutMin=[]  DifferentiatorOutMax=[]  FilterDiffOutCoefMin=[]  FilterDiffOutCoefMax=[]  ReciprocalOutMin=[]  ReciprocalOutMax=[]  SumDenOutMin=[]  SumDenOutMax=[]  SumNumOutMin=[]  SumNumOutMax=[]  DivideOutMin=[]  DivideOutMax=[]  UdiffTsProdOutMin=[]  UdiffTsProdOutMax=[]  NTsProdOutMin=[]  NTsProdOutMax=[]  UintegralTsProdOutMin=[]  UintegralTsProdOutMax=[]  UngainTsProdOutMin=[]  UngainTsProdOutMax=[]  ClampingZeroOutDataTypeStr=Inherit: Inherit via back propagation  ClampingZeroOutMin=[]  ClampingZeroOutMax=[]  FilterDenConstantOutDataTypeStr=Inherit: Inherit via back propagation  FilterDenConstantOutMin=[]  FilterDenConstantOutMax=[]  PCopyOutDataTypeStr=Inherit: Inherit via back propagation  PCopyOutMin=[]  PCopyOutMax=[]  NCopyOutDataTypeStr=Inherit: Inherit via back propagation  NCopyOutMin=[]  NCopyOutMax=[]  IntegratorContinuousStateAttributes=''  IntegratorStateMustResolveToSignalObject=off  IntegratorRTWStateStorageClass=Auto  FilterContinuousStateAttributes=''  FilterStateMustResolveToSignalObject=off  FilterRTWStateStorageClass=Auto  ParallelPVariant=InternalParameters  IdealPVariant=Disabled  IVariant=InternalParameters  DVariant=InternalParameters  IntegratorVariant=Continuous  SatVariant=Disabled  AWVariant=Passthrough  PCopyVariant=Disabled  TRVariant=Disabled  FdbkBlocksVariant=Forward  IdealPFdbkVariant=Disabled  SatFdbkVariant=Disabled  DerivativeFilterVariant=ContFilter  NVariant=InternalParameters  NCopyVariant=Disabled  FilterICVariant=InternalICsFilter  IntegratorICVariant=InternalICs  ExternalResetVariant=Disabled  TRSumVariant=Passthrough  SumFdbkVariant=Disabled  SumVariant=Sum_PID  TsampFilterVariant=InternalTs  TsampNgainVariant=Passthrough  TsampIntegralVariant=Disabled_SignalSpec  ExternalSaturationOutDataTypeStr=Inherit: Same as second input  DerivativeSourceVariant=ErrorSignal  PreIntVariant=InternalPreInt
  Saturation3 : Saturate  UpperLimit=2  LowerLimit=-2  ZeroCross=off
  T : Outport
  F : Outport  Port=2
  wires:
  MATLAB Function9/1(T) -> Saturation3/1
  PID Controller2/1 -> MATLAB Function9/1(F), F/1
  L/1 -> Minus10/1
  Phi4/1 -> MATLAB Function9/4(Phi4)
  Minus10/1 -> PID Controller2/1
  TargetL/1 -> Minus10/2
  Tp/1 -> MATLAB Function9/2(Tp)
  Phi1/1 -> MATLAB Function9/3(Phi1)
  Saturation3/1 -> T/1

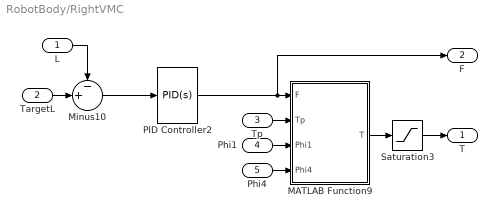
== system RobotBody/RightVMC ==
  L : Inport
  TargetL : Inport  Port=2
  Tp : Inport  Port=3
  Phi1 : Inport  Port=4
  Phi4 : Inport  Port=5
  MATLAB Function9 : MATLAB Function  TreatAsAtomicUnit=on
  Minus10 : Sum  Inputs=-+|
  PID Controller2 : slpidlib/PID Controller  Controller=PID  Form=Parallel  TimeDomain=Continuous-time  UseExternalTs=off  SampleTime=-1  IntegratorMethod=Forward Euler  FilterMethod=Forward Euler  ControllerParametersSource=internal  P=500  I=1100  UseKiTs=off  D=50  UseExternalDerivativeSource=off  N=100  UseFilter=on  TunerSelectOption=Transfer Function Based (PID Tuner App)  InitialConditionSource=internal  InitialConditionForIntegrator=0  InitialConditionForFilter=0  DifferentiatorICPrevScaledInput=0  ExternalReset=none  TrackingMode=off  Kt=1  LimitOutput=off  SatLimitsSource=internal  UpperSaturationLimit=inf  LowerSaturationLimit=-inf  LinearizeAsGain=on  AntiWindupMode=none  Kb=1  LimitIntegrator=off  UpperIntegratorSaturationLimit=inf  LowerIntegratorSaturationLimit=-inf  POutMin=[]  POutMax=[]  IOutMin=[]  IOutMax=[]  DOutMin=[]  DOutMax=[]  NOutMin=[]  NOutMax=[]  SumOutMin=[]  SumOutMax=[]  SaturationOutMin=[]  SaturationOutMax=[]  PParamMin=[]  PParamMax=[]  IParamMin=[]  IParamMax=[]  DParamMin=[]  DParamMax=[]  NParamMin=[]  NParamMax=[]  KbParamMin=[]  KbParamMax=[]  KtParamMin=[]  KtParamMax=[]  KbOutMin=[]  KbOutMax=[]  KtOutMin=[]  KtOutMax=[]  IntegratorOutMin=[]  IntegratorOutMax=[]  FilterOutMin=[]  FilterOutMax=[]  SumI1OutMin=[]  SumI1OutMax=[]  SumI2OutMin=[]  SumI2OutMax=[]  SumI3OutMin=[]  SumI3OutMax=[]  SumI4OutMin=[]  SumI4OutMax=[]  SumDOutMin=[]  SumDOutMax=[]  DifferentiatorOutMin=[]  DifferentiatorOutMax=[]  FilterDiffOutCoefMin=[]  FilterDiffOutCoefMax=[]  ReciprocalOutMin=[]  ReciprocalOutMax=[]  SumDenOutMin=[]  SumDenOutMax=[]  SumNumOutMin=[]  SumNumOutMax=[]  DivideOutMin=[]  DivideOutMax=[]  UdiffTsProdOutMin=[]  UdiffTsProdOutMax=[]  NTsProdOutMin=[]  NTsProdOutMax=[]  UintegralTsProdOutMin=[]  UintegralTsProdOutMax=[]  UngainTsProdOutMin=[]  UngainTsProdOutMax=[]  ClampingZeroOutDataTypeStr=Inherit: Inherit via back propagation  ClampingZeroOutMin=[]  ClampingZeroOutMax=[]  FilterDenConstantOutDataTypeStr=Inherit: Inherit via back propagation  FilterDenConstantOutMin=[]  FilterDenConstantOutMax=[]  PCopyOutDataTypeStr=Inherit: Inherit via back propagation  PCopyOutMin=[]  PCopyOutMax=[]  NCopyOutDataTypeStr=Inherit: Inherit via back propagation  NCopyOutMin=[]  NCopyOutMax=[]  IntegratorContinuousStateAttributes=''  IntegratorStateMustResolveToSignalObject=off  IntegratorRTWStateStorageClass=Auto  FilterContinuousStateAttributes=''  FilterStateMustResolveToSignalObject=off  FilterRTWStateStorageClass=Auto  ParallelPVariant=InternalParameters  IdealPVariant=Disabled  IVariant=InternalParameters  DVariant=InternalParameters  IntegratorVariant=Continuous  SatVariant=Disabled  AWVariant=Passthrough  PCopyVariant=Disabled  TRVariant=Disabled  FdbkBlocksVariant=Forward  IdealPFdbkVariant=Disabled  SatFdbkVariant=Disabled  DerivativeFilterVariant=ContFilter  NVariant=InternalParameters  NCopyVariant=Disabled  FilterICVariant=InternalICsFilter  IntegratorICVariant=InternalICs  ExternalResetVariant=Disabled  TRSumVariant=Passthrough  SumFdbkVariant=Disabled  SumVariant=Sum_PID  TsampFilterVariant=InternalTs  TsampNgainVariant=Passthrough  TsampIntegralVariant=Disabled_SignalSpec  ExternalSaturationOutDataTypeStr=Inherit: Same as second input  DerivativeSourceVariant=ErrorSignal  PreIntVariant=InternalPreInt
  Saturation3 : Saturate  UpperLimit=2  LowerLimit=-2  ZeroCross=off
  T : Outport
  F : Outport  Port=2
  wires:
  MATLAB Function9/1(T) -> Saturation3/1
  PID Controller2/1 -> F/1, MATLAB Function9/1(F)
  L/1 -> Minus10/1
  Phi4/1 -> MATLAB Function9/4(Phi4)
  Minus10/1 -> PID Controller2/1
  TargetL/1 -> Minus10/2
  Tp/1 -> MATLAB Function9/2(Tp)
  Phi1/1 -> MATLAB Function9/3(Phi1)
  Saturation3/1 -> T/1
